simulink model "Model_silnika2"  (R2018a)
settings: Solver=ode45  StartTime=0.0  StopTime=600  FixedStep=1  MaxStep=0.004  RelTol=1e-8  EnableMultiTasking=on
values from neighbouring files (symbols this model uses):
  G = 4.2    [net_opuznienie_30.mat]    (also in parametrySilnika.m)
  J = 1    [net_opuznienie_30.mat]    (also in parametrySilnika.m)
  Lt = 46    [net_opuznienie_30.mat]    (also in parametrySilnika.m)
  Lw = 125    [net_opuznienie_30.mat]    (also in parametrySilnika.m)
  Rt = 5    [net_opuznienie_30.mat]    (also in parametrySilnika.m)
undefined symbols (not defined in the file or in its folder): sigbuilder_block
libraries: neural x22, simulink x2
(part 2 of 3)

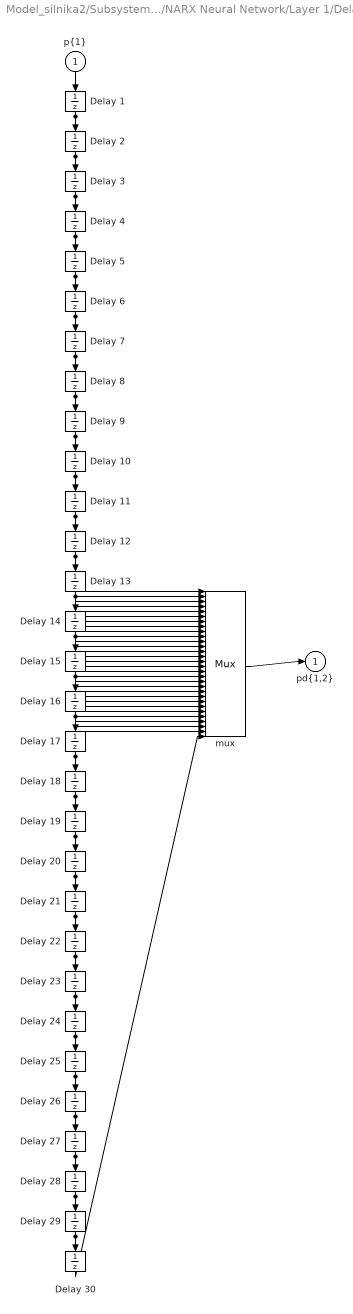
== system Model_silnika2/Subsystem/NARX Neural Network/Layer 1/Delays 2 ==
  "p{1}" : Inport  PortDimensions=3  SampleTime=0.1
      mask Display: e = 0.06;c1 = [120 230 180]/255;c2 = ([120 230 180]+0)/(256+128);c3 = ([120 230 180]+128)/(256+128);patch([0 1 1 0],[0 0 1 1],c1);patch([0 1 1 1-e 1-e 0+e],[0 0 1 1-e 0+e 0+e],c2);patch([0 0 1 1-e 0+e 0+e],[0 1 1 1-e 1-e 0+e],c3);plot([0 1 1 0 0],[0 0 1 1 0]);
  Delay 1 : UnitDelay  InitialCondition=pi_input_2_delayed_1  SampleTime=0.1
      mask Display: e = 0.06;c1 = [120 150 230]/255;c2 = ([120 150 230]+0)/383;c3 = ([120 150 230]+128)/383;patch([0 1 1 0],[0 0 1 1],c1);patch([0 1 1 1-e 1-e 0+e],[0 0 1 1-e 0+e 0+e],c2);patch([0 0 1 1-e 0+e 0+e],[0 1 1 1-e 1-e 0+e],c3);plot([0 1 1 0 0],[0 0 1 1 0]);disp('D')
  Delay 10 : UnitDelay  InitialCondition=pi_input_2_delayed_10  SampleTime=0.1
      mask Display: e = 0.06;c1 = [120 150 230]/255;c2 = ([120 150 230]+0)/383;c3 = ([120 150 230]+128)/383;patch([0 1 1 0],[0 0 1 1],c1);patch([0 1 1 1-e 1-e 0+e],[0 0 1 1-e 0+e 0+e],c2);patch([0 0 1 1-e 0+e 0+e],[0 1 1 1-e 1-e 0+e],c3);plot([0 1 1 0 0],[0 0 1 1 0]);disp('D')
  Delay 11 : UnitDelay  InitialCondition=pi_input_2_delayed_11  SampleTime=0.1
      mask Display: e = 0.06;c1 = [120 150 230]/255;c2 = ([120 150 230]+0)/383;c3 = ([120 150 230]+128)/383;patch([0 1 1 0],[0 0 1 1],c1);patch([0 1 1 1-e 1-e 0+e],[0 0 1 1-e 0+e 0+e],c2);patch([0 0 1 1-e 0+e 0+e],[0 1 1 1-e 1-e 0+e],c3);plot([0 1 1 0 0],[0 0 1 1 0]);disp('D')
  Delay 12 : UnitDelay  InitialCondition=pi_input_2_delayed_12  SampleTime=0.1
      mask Display: e = 0.06;c1 = [120 150 230]/255;c2 = ([120 150 230]+0)/383;c3 = ([120 150 230]+128)/383;patch([0 1 1 0],[0 0 1 1],c1);patch([0 1 1 1-e 1-e 0+e],[0 0 1 1-e 0+e 0+e],c2);patch([0 0 1 1-e 0+e 0+e],[0 1 1 1-e 1-e 0+e],c3);plot([0 1 1 0 0],[0 0 1 1 0]);disp('D')
  Delay 13 : UnitDelay  InitialCondition=pi_input_2_delayed_13  SampleTime=0.1
      mask Display: e = 0.06;c1 = [120 150 230]/255;c2 = ([120 150 230]+0)/383;c3 = ([120 150 230]+128)/383;patch([0 1 1 0],[0 0 1 1],c1);patch([0 1 1 1-e 1-e 0+e],[0 0 1 1-e 0+e 0+e],c2);patch([0 0 1 1-e 0+e 0+e],[0 1 1 1-e 1-e 0+e],c3);plot([0 1 1 0 0],[0 0 1 1 0]);disp('D')
  Delay 14 : UnitDelay  InitialCondition=pi_input_2_delayed_14  SampleTime=0.1
      mask Display: e = 0.06;c1 = [120 150 230]/255;c2 = ([120 150 230]+0)/383;c3 = ([120 150 230]+128)/383;patch([0 1 1 0],[0 0 1 1],c1);patch([0 1 1 1-e 1-e 0+e],[0 0 1 1-e 0+e 0+e],c2);patch([0 0 1 1-e 0+e 0+e],[0 1 1 1-e 1-e 0+e],c3);plot([0 1 1 0 0],[0 0 1 1 0]);disp('D')
  Delay 15 : UnitDelay  InitialCondition=pi_input_2_delayed_15  SampleTime=0.1
      mask Display: e = 0.06;c1 = [120 150 230]/255;c2 = ([120 150 230]+0)/383;c3 = ([120 150 230]+128)/383;patch([0 1 1 0],[0 0 1 1],c1);patch([0 1 1 1-e 1-e 0+e],[0 0 1 1-e 0+e 0+e],c2);patch([0 0 1 1-e 0+e 0+e],[0 1 1 1-e 1-e 0+e],c3);plot([0 1 1 0 0],[0 0 1 1 0]);disp('D')
  Delay 16 : UnitDelay  InitialCondition=pi_input_2_delayed_16  SampleTime=0.1
      mask Display: e = 0.06;c1 = [120 150 230]/255;c2 = ([120 150 230]+0)/383;c3 = ([120 150 230]+128)/383;patch([0 1 1 0],[0 0 1 1],c1);patch([0 1 1 1-e 1-e 0+e],[0 0 1 1-e 0+e 0+e],c2);patch([0 0 1 1-e 0+e 0+e],[0 1 1 1-e 1-e 0+e],c3);plot([0 1 1 0 0],[0 0 1 1 0]);disp('D')
  Delay 17 : UnitDelay  InitialCondition=pi_input_2_delayed_17  SampleTime=0.1
      mask Display: e = 0.06;c1 = [120 150 230]/255;c2 = ([120 150 230]+0)/383;c3 = ([120 150 230]+128)/383;patch([0 1 1 0],[0 0 1 1],c1);patch([0 1 1 1-e 1-e 0+e],[0 0 1 1-e 0+e 0+e],c2);patch([0 0 1 1-e 0+e 0+e],[0 1 1 1-e 1-e 0+e],c3);plot([0 1 1 0 0],[0 0 1 1 0]);disp('D')
  Delay 18 : UnitDelay  InitialCondition=pi_input_2_delayed_18  SampleTime=0.1
      mask Display: e = 0.06;c1 = [120 150 230]/255;c2 = ([120 150 230]+0)/383;c3 = ([120 150 230]+128)/383;patch([0 1 1 0],[0 0 1 1],c1);patch([0 1 1 1-e 1-e 0+e],[0 0 1 1-e 0+e 0+e],c2);patch([0 0 1 1-e 0+e 0+e],[0 1 1 1-e 1-e 0+e],c3);plot([0 1 1 0 0],[0 0 1 1 0]);disp('D')
  Delay 19 : UnitDelay  InitialCondition=pi_input_2_delayed_19  SampleTime=0.1
      mask Display: e = 0.06;c1 = [120 150 230]/255;c2 = ([120 150 230]+0)/383;c3 = ([120 150 230]+128)/383;patch([0 1 1 0],[0 0 1 1],c1);patch([0 1 1 1-e 1-e 0+e],[0 0 1 1-e 0+e 0+e],c2);patch([0 0 1 1-e 0+e 0+e],[0 1 1 1-e 1-e 0+e],c3);plot([0 1 1 0 0],[0 0 1 1 0]);disp('D')
  Delay 2 : UnitDelay  InitialCondition=pi_input_2_delayed_2  SampleTime=0.1
      mask Display: e = 0.06;c1 = [120 150 230]/255;c2 = ([120 150 230]+0)/383;c3 = ([120 150 230]+128)/383;patch([0 1 1 0],[0 0 1 1],c1);patch([0 1 1 1-e 1-e 0+e],[0 0 1 1-e 0+e 0+e],c2);patch([0 0 1 1-e 0+e 0+e],[0 1 1 1-e 1-e 0+e],c3);plot([0 1 1 0 0],[0 0 1 1 0]);disp('D')
  Delay 20 : UnitDelay  InitialCondition=pi_input_2_delayed_20  SampleTime=0.1
      mask Display: e = 0.06;c1 = [120 150 230]/255;c2 = ([120 150 230]+0)/383;c3 = ([120 150 230]+128)/383;patch([0 1 1 0],[0 0 1 1],c1);patch([0 1 1 1-e 1-e 0+e],[0 0 1 1-e 0+e 0+e],c2);patch([0 0 1 1-e 0+e 0+e],[0 1 1 1-e 1-e 0+e],c3);plot([0 1 1 0 0],[0 0 1 1 0]);disp('D')
  Delay 21 : UnitDelay  InitialCondition=pi_input_2_delayed_21  SampleTime=0.1
      mask Display: e = 0.06;c1 = [120 150 230]/255;c2 = ([120 150 230]+0)/383;c3 = ([120 150 230]+128)/383;patch([0 1 1 0],[0 0 1 1],c1);patch([0 1 1 1-e 1-e 0+e],[0 0 1 1-e 0+e 0+e],c2);patch([0 0 1 1-e 0+e 0+e],[0 1 1 1-e 1-e 0+e],c3);plot([0 1 1 0 0],[0 0 1 1 0]);disp('D')
  Delay 22 : UnitDelay  InitialCondition=pi_input_2_delayed_22  SampleTime=0.1
      mask Display: e = 0.06;c1 = [120 150 230]/255;c2 = ([120 150 230]+0)/383;c3 = ([120 150 230]+128)/383;patch([0 1 1 0],[0 0 1 1],c1);patch([0 1 1 1-e 1-e 0+e],[0 0 1 1-e 0+e 0+e],c2);patch([0 0 1 1-e 0+e 0+e],[0 1 1 1-e 1-e 0+e],c3);plot([0 1 1 0 0],[0 0 1 1 0]);disp('D')
  Delay 23 : UnitDelay  InitialCondition=pi_input_2_delayed_23  SampleTime=0.1
      mask Display: e = 0.06;c1 = [120 150 230]/255;c2 = ([120 150 230]+0)/383;c3 = ([120 150 230]+128)/383;patch([0 1 1 0],[0 0 1 1],c1);patch([0 1 1 1-e 1-e 0+e],[0 0 1 1-e 0+e 0+e],c2);patch([0 0 1 1-e 0+e 0+e],[0 1 1 1-e 1-e 0+e],c3);plot([0 1 1 0 0],[0 0 1 1 0]);disp('D')
  Delay 24 : UnitDelay  InitialCondition=pi_input_2_delayed_24  SampleTime=0.1
      mask Display: e = 0.06;c1 = [120 150 230]/255;c2 = ([120 150 230]+0)/383;c3 = ([120 150 230]+128)/383;patch([0 1 1 0],[0 0 1 1],c1);patch([0 1 1 1-e 1-e 0+e],[0 0 1 1-e 0+e 0+e],c2);patch([0 0 1 1-e 0+e 0+e],[0 1 1 1-e 1-e 0+e],c3);plot([0 1 1 0 0],[0 0 1 1 0]);disp('D')
  Delay 25 : UnitDelay  InitialCondition=pi_input_2_delayed_25  SampleTime=0.1
      mask Display: e = 0.06;c1 = [120 150 230]/255;c2 = ([120 150 230]+0)/383;c3 = ([120 150 230]+128)/383;patch([0 1 1 0],[0 0 1 1],c1);patch([0 1 1 1-e 1-e 0+e],[0 0 1 1-e 0+e 0+e],c2);patch([0 0 1 1-e 0+e 0+e],[0 1 1 1-e 1-e 0+e],c3);plot([0 1 1 0 0],[0 0 1 1 0]);disp('D')
  Delay 26 : UnitDelay  InitialCondition=pi_input_2_delayed_26  SampleTime=0.1
      mask Display: e = 0.06;c1 = [120 150 230]/255;c2 = ([120 150 230]+0)/383;c3 = ([120 150 230]+128)/383;patch([0 1 1 0],[0 0 1 1],c1);patch([0 1 1 1-e 1-e 0+e],[0 0 1 1-e 0+e 0+e],c2);patch([0 0 1 1-e 0+e 0+e],[0 1 1 1-e 1-e 0+e],c3);plot([0 1 1 0 0],[0 0 1 1 0]);disp('D')
  Delay 27 : UnitDelay  InitialCondition=pi_input_2_delayed_27  SampleTime=0.1
      mask Display: e = 0.06;c1 = [120 150 230]/255;c2 = ([120 150 230]+0)/383;c3 = ([120 150 230]+128)/383;patch([0 1 1 0],[0 0 1 1],c1);patch([0 1 1 1-e 1-e 0+e],[0 0 1 1-e 0+e 0+e],c2);patch([0 0 1 1-e 0+e 0+e],[0 1 1 1-e 1-e 0+e],c3);plot([0 1 1 0 0],[0 0 1 1 0]);disp('D')
  Delay 28 : UnitDelay  InitialCondition=pi_input_2_delayed_28  SampleTime=0.1
      mask Display: e = 0.06;c1 = [120 150 230]/255;c2 = ([120 150 230]+0)/383;c3 = ([120 150 230]+128)/383;patch([0 1 1 0],[0 0 1 1],c1);patch([0 1 1 1-e 1-e 0+e],[0 0 1 1-e 0+e 0+e],c2);patch([0 0 1 1-e 0+e 0+e],[0 1 1 1-e 1-e 0+e],c3);plot([0 1 1 0 0],[0 0 1 1 0]);disp('D')
  Delay 29 : UnitDelay  InitialCondition=pi_input_2_delayed_29  SampleTime=0.1
      mask Display: e = 0.06;c1 = [120 150 230]/255;c2 = ([120 150 230]+0)/383;c3 = ([120 150 230]+128)/383;patch([0 1 1 0],[0 0 1 1],c1);patch([0 1 1 1-e 1-e 0+e],[0 0 1 1-e 0+e 0+e],c2);patch([0 0 1 1-e 0+e 0+e],[0 1 1 1-e 1-e 0+e],c3);plot([0 1 1 0 0],[0 0 1 1 0]);disp('D')
  Delay 3 : UnitDelay  InitialCondition=pi_input_2_delayed_3  SampleTime=0.1
      mask Display: e = 0.06;c1 = [120 150 230]/255;c2 = ([120 150 230]+0)/383;c3 = ([120 150 230]+128)/383;patch([0 1 1 0],[0 0 1 1],c1);patch([0 1 1 1-e 1-e 0+e],[0 0 1 1-e 0+e 0+e],c2);patch([0 0 1 1-e 0+e 0+e],[0 1 1 1-e 1-e 0+e],c3);plot([0 1 1 0 0],[0 0 1 1 0]);disp('D')
  Delay 30 : UnitDelay  InitialCondition=pi_input_2_delayed_30  SampleTime=0.1
      mask Display: e = 0.06;c1 = [120 150 230]/255;c2 = ([120 150 230]+0)/383;c3 = ([120 150 230]+128)/383;patch([0 1 1 0],[0 0 1 1],c1);patch([0 1 1 1-e 1-e 0+e],[0 0 1 1-e 0+e 0+e],c2);patch([0 0 1 1-e 0+e 0+e],[0 1 1 1-e 1-e 0+e],c3);plot([0 1 1 0 0],[0 0 1 1 0]);disp('D')
  Delay 4 : UnitDelay  InitialCondition=pi_input_2_delayed_4  SampleTime=0.1
      mask Display: e = 0.06;c1 = [120 150 230]/255;c2 = ([120 150 230]+0)/383;c3 = ([120 150 230]+128)/383;patch([0 1 1 0],[0 0 1 1],c1);patch([0 1 1 1-e 1-e 0+e],[0 0 1 1-e 0+e 0+e],c2);patch([0 0 1 1-e 0+e 0+e],[0 1 1 1-e 1-e 0+e],c3);plot([0 1 1 0 0],[0 0 1 1 0]);disp('D')
  Delay 5 : UnitDelay  InitialCondition=pi_input_2_delayed_5  SampleTime=0.1
      mask Display: e = 0.06;c1 = [120 150 230]/255;c2 = ([120 150 230]+0)/383;c3 = ([120 150 230]+128)/383;patch([0 1 1 0],[0 0 1 1],c1);patch([0 1 1 1-e 1-e 0+e],[0 0 1 1-e 0+e 0+e],c2);patch([0 0 1 1-e 0+e 0+e],[0 1 1 1-e 1-e 0+e],c3);plot([0 1 1 0 0],[0 0 1 1 0]);disp('D')
  Delay 6 : UnitDelay  InitialCondition=pi_input_2_delayed_6  SampleTime=0.1
      mask Display: e = 0.06;c1 = [120 150 230]/255;c2 = ([120 150 230]+0)/383;c3 = ([120 150 230]+128)/383;patch([0 1 1 0],[0 0 1 1],c1);patch([0 1 1 1-e 1-e 0+e],[0 0 1 1-e 0+e 0+e],c2);patch([0 0 1 1-e 0+e 0+e],[0 1 1 1-e 1-e 0+e],c3);plot([0 1 1 0 0],[0 0 1 1 0]);disp('D')
  Delay 7 : UnitDelay  InitialCondition=pi_input_2_delayed_7  SampleTime=0.1
      mask Display: e = 0.06;c1 = [120 150 230]/255;c2 = ([120 150 230]+0)/383;c3 = ([120 150 230]+128)/383;patch([0 1 1 0],[0 0 1 1],c1);patch([0 1 1 1-e 1-e 0+e],[0 0 1 1-e 0+e 0+e],c2);patch([0 0 1 1-e 0+e 0+e],[0 1 1 1-e 1-e 0+e],c3);plot([0 1 1 0 0],[0 0 1 1 0]);disp('D')
  Delay 8 : UnitDelay  InitialCondition=pi_input_2_delayed_8  SampleTime=0.1
      mask Display: e = 0.06;c1 = [120 150 230]/255;c2 = ([120 150 230]+0)/383;c3 = ([120 150 230]+128)/383;patch([0 1 1 0],[0 0 1 1],c1);patch([0 1 1 1-e 1-e 0+e],[0 0 1 1-e 0+e 0+e],c2);patch([0 0 1 1-e 0+e 0+e],[0 1 1 1-e 1-e 0+e],c3);plot([0 1 1 0 0],[0 0 1 1 0]);disp('D')
  Delay 9 : UnitDelay  InitialCondition=pi_input_2_delayed_9  SampleTime=0.1
      mask Display: e = 0.06;c1 = [120 150 230]/255;c2 = ([120 150 230]+0)/383;c3 = ([120 150 230]+128)/383;patch([0 1 1 0],[0 0 1 1],c1);patch([0 1 1 1-e 1-e 0+e],[0 0 1 1-e 0+e 0+e],c2);patch([0 0 1 1-e 0+e 0+e],[0 1 1 1-e 1-e 0+e],c3);plot([0 1 1 0 0],[0 0 1 1 0]);disp('D')
  mux : Mux  Inputs=30
      mask Display: e = 0.06;c1 = [120 150 230]/255;c2 = ([120 150 230]+0)/383;c3 = ([120 150 230]+128)/383;patch([0 1 1 0],[0 0 1 1],c1);patch([0 1 1 1-e 1-e 0+e],[0 0 1 1-e 0+e 0+e],c2);patch([0 0 1 1-e 0+e 0+e],[0 1 1 1-e 1-e 0+e],c3);plot([0 1 1 0 0],[0 0 1 1 0]);disp('Mux')
  "pd{1,2}" : Outport
      mask Display: e = 0.06;c1 = [120 230 180]/255;c2 = ([120 230 180]+0)/(256+128);c3 = ([120 230 180]+128)/(256+128);patch([0 1 1 0],[0 0 1 1],c1);patch([0 1 1 1-e 1-e 0+e],[0 0 1 1-e 0+e 0+e],c2);patch([0 0 1 1-e 0+e 0+e],[0 1 1 1-e 1-e 0+e],c3);plot([0 1 1 0 0],[0 0 1 1 0]);
  wires:
  "p{1}"/1 -> Delay 1/1
  Delay 1/1 -> Delay 2/1, mux/1
  Delay 2/1 -> Delay 3/1, mux/2
  Delay 3/1 -> Delay 4/1, mux/3
  Delay 4/1 -> Delay 5/1, mux/4
  Delay 5/1 -> Delay 6/1, mux/5
  Delay 6/1 -> Delay 7/1, mux/6
  Delay 7/1 -> Delay 8/1, mux/7
  Delay 8/1 -> Delay 9/1, mux/8
  Delay 9/1 -> Delay 10/1, mux/9
  Delay 10/1 -> Delay 11/1, mux/10
  Delay 11/1 -> Delay 12/1, mux/11
  Delay 12/1 -> Delay 13/1, mux/12
  Delay 13/1 -> Delay 14/1, mux/13
  Delay 14/1 -> Delay 15/1, mux/14
  Delay 15/1 -> Delay 16/1, mux/15
  Delay 16/1 -> Delay 17/1, mux/16
  Delay 17/1 -> Delay 18/1, mux/17
  Delay 18/1 -> Delay 19/1, mux/18
  Delay 19/1 -> Delay 20/1, mux/19
  Delay 20/1 -> Delay 21/1, mux/20
  Delay 21/1 -> Delay 22/1, mux/21
  Delay 22/1 -> Delay 23/1, mux/22
  Delay 23/1 -> Delay 24/1, mux/23
  Delay 24/1 -> Delay 25/1, mux/24
  Delay 25/1 -> Delay 26/1, mux/25
  Delay 26/1 -> Delay 27/1, mux/26
  Delay 27/1 -> Delay 28/1, mux/27
  Delay 28/1 -> Delay 29/1, mux/28
  Delay 29/1 -> Delay 30/1, mux/29
  Delay 30/1 -> mux/30
  mux/1 -> "pd{1,2}"/1

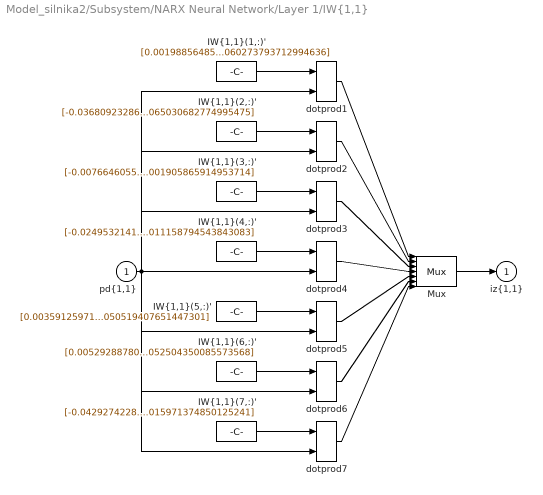
== system Model_silnika2/Subsystem/NARX Neural Network/Layer 1/IW{1,1} ==
  "pd{1,1}" : Inport  PortDimensions=93  SampleTime=0.1
      mask Display: e = 0.06;c1 = [120 230 180]/255;c2 = ([120 230 180]+0)/(256+128);c3 = ([120 230 180]+128)/(256+128);patch([0 1 1 0],[0 0 1 1],c1);patch([0 1 1 1-e 1-e 0+e],[0 0 1 1-e 0+e 0+e],c2);patch([0 0 1 1-e 0+e 0+e],[0 1 1 1-e 1-e 0+e],c3);plot([0 1 1 0 0],[0 0 1 1 0]);
  "IW{1,1}(1,:)'" : Constant  Value=[0.0019885648572870711;0.00017353216044262241;0.00020246318392944663;0.0012877889136962829;0.0041621575399698862;0.004146431914045119;0.0031122554266859951;0.0072578529035021563;0.007221608539589231;0.0052886978249656455;0.0096265541469795594;0.0096097866153640188;0.0037072305592038514;0.010159213000665725;0.010153021947951481;0.0020284555667614071;0.0094199191911381822;0.0094369659993983907;0.0022816816539381404;0.0071232650382990906;0.0071537518067209304;0.0016626187475556919;0.0047518269829249444;0.0047531056147696706;0.0020121305033980598;0.0025672373543122948;0.002577118947758473;0.0034272863518573196;0.00016888799192580465;0.00018905384494078149;0.0037618836764962589;-0.0018604907625631168;-0.0018757218477068655;0.0067485305203867987;-0.0033535570623899873;-0.0033435156926478133;0.0064292299509081932;-0.0049475392854431534;-0.0049515590045061068;0.0091330520987752805;-0.0058607117799318615;-0.0058645572190691719;0.0097185636515801262;-0.0063177974309289201;-0.0062841625672411484;0.011049853079969906;-0.0066066019753691129;-0.00660886754201713;0.011639652187494744;-0.0058638683193952866;-0.0058674765812183555;0.012277307839238506;-0.0062434092143199308;-0.006223173999384257;0.012184300722183823;-0.0049910581364777896;-0.0049602741139057847;0.012369523833305114;-0.0040177057475507556;-0.0040258670882894884;0.012707114686688135;-0.0031374496005083527;-0.0031135632071982462;0.01199815190430247;-0.0014803465930950306;-0.0014817157917846025;0.011745661192756328;-0.00013594683155318063;-0.00012740864850212361;0.012929416864156986;0.00094004208381961172;0.00096521495097527221;0.012502965348679465;0.0023279754869333273;0.0023414545896575357;0.012482435998225856;0.0035419671709262944;0.0035762178877970798;0.011934548300930431;0.0053325738868501282;0.0053320827850480155;0.013046636614108929;0.0062096453902115182;0.0062246560250742529;0.011663539355452375;0.0064304649638875439;0.0064084155992088186;0.010450554421592198;0.0061677203783633708;0.0061797856121988005;0.011067516086346763;0.0060248674964442734;0.0060273793712994636]
      mask Display: e = 0.06;c1 = [120 150 230]/255;c2 = ([120 150 230]+0)/383;c3 = ([120 150 230]+128)/383;patch([0 1 1 0],[0 0 1 1],c1);patch([0 1 1 1-e 1-e 0+e],[0 0 1 1-e 0+e 0+e],c2);patch([0 0 1 1-e 0+e 0+e],[0 1 1 1-e 1-e 0+e],c3);plot([0 1 1 0 0],[0 0 1 1 0]);disp('Weights');
  "IW{1,1}(2,:)'" : Constant  Value=[-0.03680923286623293;0.025215958210341321;0.025191876987067676;-0.034153384448485612;0.024063629556723632;0.02404265159227895;-0.030487212660508366;0.022144925280749239;0.022106187781516771;-0.026859037089298522;0.019689245268806482;0.019715780530329522;-0.02468526855312566;0.016516588171180301;0.016524213109626922;-0.022695789377278296;0.012715426366594689;0.012752544524029415;-0.020156834591642563;0.0083737663442279859;0.008377356952699113;-0.01792882104581392;0.003963595507632851;0.0039637470964308946;-0.01498767046199004;-4.9456871022110553e-05;-7.9445729385161992e-05;-0.011372105946886809;-0.0035765479627977502;-0.0035923381340926702;-0.0079894622040690734;-0.0066533549247146948;-0.0066203605988653397;-0.004043202763429384;-0.0089192912789356742;-0.0088909998267149709;-0.001375045309514116;-0.011229821222691011;-0.011233430056455107;0.0020227825901768999;-0.012859892709453988;-0.012861008152047815;0.0048546825941336831;-0.01383926836744738;-0.013829553396572589;0.0072545813229751262;-0.014533696655662112;-0.014547831275745167;0.0089438640831206399;-0.01445291075726691;-0.014456316411346329;0.010370767359619755;-0.014669870337057684;-0.014666959249565592;0.011051647416366481;-0.013851038859060147;-0.013854928157819064;0.011414804606182162;-0.013440498542700576;-0.013437280320999244;0.011817958426225416;-0.013077862131358578;-0.013085944535545744;0.011889264426307739;-0.012151921817595127;-0.012152494578213956;0.011803270873627833;-0.011293556937451647;-0.011270072938144112;0.011858328407325773;-0.010430807682652582;-0.010431336347693823;0.011339670981287958;-0.0094576249475570254;-0.0094426100981729894;0.011057000374518903;-0.0086155962492994662;-0.0086540404890446624;0.0099484260683701687;-0.0076154062550492672;-0.007594172765159223;0.009014773366731399;-0.0069859248919153065;-0.0069986384129998701;0.0066053208315398244;-0.0067985909291236029;-0.0067978012725416559;0.0044751367755976202;-0.0067350110232024911;-0.0067473465466301886;0.0041511708943185247;-0.006514042265822589;-0.0065030682774995475]
      mask Display: e = 0.06;c1 = [120 150 230]/255;c2 = ([120 150 230]+0)/383;c3 = ([120 150 230]+128)/383;patch([0 1 1 0],[0 0 1 1],c1);patch([0 1 1 1-e 1-e 0+e],[0 0 1 1-e 0+e 0+e],c2);patch([0 0 1 1-e 0+e 0+e],[0 1 1 1-e 1-e 0+e],c3);plot([0 1 1 0 0],[0 0 1 1 0]);disp('Weights');
  "IW{1,1}(3,:)'" : Constant  Value=[-0.0076646055777691447;0.0070763234502732838;0.0070842203536176764;-0.004594913111176613;0.00038964116521432435;0.00041137158750551158;-0.0055103091263933625;-0.0049698101367087431;-0.0049412877899630211;-0.0075325442099127291;-0.0095426577629565013;-0.0095450227927753265;-0.0060297870176984304;-0.01209467695642937;-0.012105590036045317;-0.0044564633847823439;-0.012815090396055499;-0.012833693489322106;-0.0050632626749825185;-0.011506247072813098;-0.011504150966507259;-0.0041971286806833982;-0.0099695988637943291;-0.0099425354167575215;-0.0047297180263328863;-0.0082225182406181346;-0.0082109420612531767;-0.0067358883907070741;-0.0059865998064806223;-0.0059684859614520733;-0.0074868297025780604;-0.0040227287991187544;-0.0040515110992039843;-0.011732321752348762;-0.002409628897517291;-0.0024049134196149312;-0.012627903895818169;-0.00053672640906698055;-0.0005716310236179667;-0.016835849365649313;0.00086902971839981815;0.00087478298754549986;-0.018940044323451959;0.0017801611802645415;0.0018173051495409172;-0.02200354703831504;0.0025552877957088988;0.002585355729384693;-0.024609533244623949;0.0024114075415604687;0.0023826032603090465;-0.027037040480159313;0.0035213804790525938;0.0035144012931958468;-0.028721304805968094;0.0029288786376778907;0.0029422387894351893;-0.030291298317651628;0.0028880625472197555;0.0028814799615048377;-0.032013383924733345;0.00300445969541639;0.0030064049406744548;-0.031671424258573944;0.0022868466292456638;0.0023006048521897796;-0.031286120167063426;0.0017743262488769227;0.001774390100282909;-0.031572071293566019;0.0013442866037685151;0.0013360455361241812;-0.030039011394857935;0.00067713247476120387;0.0006818199996063125;-0.02884953861886283;0.00018619370936413836;0.00018991909697096154;-0.026606256381875752;-0.00086325294604902277;-0.00083595550254723428;-0.026549482570305025;-0.0010631146031886639;-0.0010670006856293985;-0.024506533022186059;-0.00043396403427776043;-0.00043993942798726393;-0.023857218832608072;0.00077160857113643981;0.00076178553565276071;-0.027315974330495405;0.0019114969343765071;0.001905865914953714]
      mask Display: e = 0.06;c1 = [120 150 230]/255;c2 = ([120 150 230]+0)/383;c3 = ([120 150 230]+128)/383;patch([0 1 1 0],[0 0 1 1],c1);patch([0 1 1 1-e 1-e 0+e],[0 0 1 1-e 0+e 0+e],c2);patch([0 0 1 1-e 0+e 0+e],[0 1 1 1-e 1-e 0+e],c3);plot([0 1 1 0 0],[0 0 1 1 0]);disp('Weights');
  "IW{1,1}(4,:)'" : Constant  Value=[-0.024953214152112446;0.017578647700541843;0.017608634271546918;-0.025588820938720846;0.014549255924575141;0.014550126941371457;-0.026417842514427088;0.01147470305506669;0.011445717308638288;-0.026961255328549059;0.0082363745066816631;0.0082013756291282516;-0.027018906125422449;0.005036783567107927;0.0050678034015124015;-0.026671111694633067;0.0022447302008953103;0.0022171969117303798;-0.026090237135677489;-0.00017533098161182927;-0.00019018529225397281;-0.025134837113502468;-0.0024871079659541965;-0.0024828696492451936;-0.023782095946141415;-0.004256367260575834;-0.0042656632777644124;-0.022130683470411014;-0.0053444351789336889;-0.005366701687299873;-0.020277090535669787;-0.0061031946592581916;-0.0060891997791776139;-0.018839830214806216;-0.006223231525543332;-0.0062156093638447672;-0.017268371700014457;-0.0062377253661623742;-0.0062643243250359642;-0.01625675960138679;-0.0057526015649238208;-0.0057310847803064627;-0.015211110193193092;-0.0049240319469992643;-0.0049306795812584748;-0.01463586456630382;-0.0039976779854303066;-0.0040410249695505595;-0.014635588838467288;-0.0028053020014475534;-0.0027980922398539877;-0.014750113931144775;-0.0015177271525010441;-0.0014799942746023087;-0.015234792103127927;-0.00010261601384378528;-8.7029409396311919e-05;-0.015998182674261625;0.0011597321065536339;0.001143829433398573;-0.016649131067453686;0.0022598269028675584;0.0022387278018720495;-0.016732540974371306;0.0033678647677113948;0.003376795470470398;-0.016903766148265997;0.0043405711349634116;0.0043066270239116595;-0.016981130992204024;0.0051828859263470788;0.0051571659249885909;-0.01664508850628334;0.0060185665848738685;0.0060070480999806523;-0.016048505280874117;0.0067545034454371908;0.0067220477720790414;-0.015167167099549997;0.0075096471932779687;0.0074816815870082489;-0.01427165616158326;0.008121188999079855;0.0081210376691659963;-0.01301693526491484;0.0088954088064422867;0.008884273434918705;-0.011429650812850183;0.0098725597150395843;0.0098790844536994563;-0.0099670414762932959;0.011129666809469901;0.011158794543843083]
      mask Display: e = 0.06;c1 = [120 150 230]/255;c2 = ([120 150 230]+0)/383;c3 = ([120 150 230]+128)/383;patch([0 1 1 0],[0 0 1 1],c1);patch([0 1 1 1-e 1-e 0+e],[0 0 1 1-e 0+e 0+e],c2);patch([0 0 1 1-e 0+e 0+e],[0 1 1 1-e 1-e 0+e],c3);plot([0 1 1 0 0],[0 0 1 1 0]);disp('Weights');
  "IW{1,1}(5,:)'" : Constant  Value=[0.0035912597198759478;0.0022194699294250204;0.0022070743640280372;0.00077847037868036687;0.0050083939769279264;0.0050228843958537196;-0.00025144755070802613;0.0071198457217213169;0.0071415387697813327;-0.00086180715771119287;0.0087201391749727984;0.0087414817602086588;-0.0031340365905234624;0.0092886883037458876;0.0092873220168890082;-0.0052954704366534296;0.0088471957109749807;0.0088259433338954574;-0.0065829532588685333;0.0072713864638687276;0.0072987417680781368;-0.0083163026255622594;0.0055368028928486843;0.0055199532455692518;-0.0097112289078713759;0.0035529734453227432;0.0035518652840302524;-0.010591020446259088;0.0013446741432513892;0.0013416992132362008;-0.011913605031789351;-0.0007186430117100544;-0.00071908121405710667;-0.011919892468382548;-0.0025882079972884874;-0.0025620137884845794;-0.013590094113028929;-0.0045526144512863503;-0.0045560491431301522;-0.013689563681360661;-0.0061740946442150283;-0.0061594999080722447;-0.014656779881288169;-0.0073538128567747956;-0.0073736306015660513;-0.015263638500944492;-0.0083611992289845533;-0.0083598034601088615;-0.015908944896438883;-0.0086414553497181565;-0.0086474989103364642;-0.016518718019227187;-0.0093603927472191498;-0.0093492063584030456;-0.017515304931307096;-0.0089816009426515013;-0.0089807669944180959;-0.018270911741919794;-0.0087790443042900703;-0.0087976678334840894;-0.01906235024901845;-0.008437788654195073;-0.0084384877720136888;-0.020472522250278725;-0.0074866456040048792;-0.0074933545891612847;-0.021479409476140545;-0.0064436338273677089;-0.0064192896558623843;-0.021732519527068981;-0.0051706023148107875;-0.0051875565808949852;-0.02259147221813064;-0.0037285928810473321;-0.0037182858034055443;-0.022650667293692871;-0.002192345434636608;-0.0022154630191904448;-0.023094601281733965;-0.00030963508331347282;-0.00028814305386080816;-0.021641636092181626;0.0013783285511740138;0.0014080306509820042;-0.020295486602463327;0.0027711832781927449;0.0027738717342319585;-0.016661812474125567;0.0038592662976353266;0.0038360091476565554;-0.0094662188722694392;0.0050267142573103335;0.0050519407651447301]
      mask Display: e = 0.06;c1 = [120 150 230]/255;c2 = ([120 150 230]+0)/383;c3 = ([120 150 230]+128)/383;patch([0 1 1 0],[0 0 1 1],c1);patch([0 1 1 1-e 1-e 0+e],[0 0 1 1-e 0+e 0+e],c2);patch([0 0 1 1-e 0+e 0+e],[0 1 1 1-e 1-e 0+e],c3);plot([0 1 1 0 0],[0 0 1 1 0]);disp('Weights');
  "IW{1,1}(6,:)'" : Constant  Value=[0.0052928878042780179;-0.0025753065097767853;-0.0025758051208712982;0.0068216665336466335;-0.0079511153434142293;-0.0079433138774494243;0.0057078495493609101;-0.012378658652655227;-0.012380743639209468;0.0046156340450630457;-0.016201851560737147;-0.01618743605339705;0.0078831837590174064;-0.018081756866652567;-0.01809827946408011;0.01159934545123035;-0.01847763344280005;-0.018473405265828382;0.013252498379862403;-0.017023380212477499;-0.017009733701925836;0.015914720827213152;-0.015412720805715483;-0.01543395358124736;0.017600574172222341;-0.013764240450822685;-0.013745752509640127;0.018193904364199202;-0.011563353566653084;-0.011538393863117875;0.019820170980550941;-0.0095168443909042361;-0.0095238984037360214;0.018449227249202713;-0.0077115338489178609;-0.0076874922431354586;0.020459729419441457;-0.005676412874902205;-0.0056893160741749559;0.018826627784329506;-0.0040012520828199517;-0.0040162515145911893;0.019173271711041266;-0.0026821762790689061;-0.0027130496675827902;0.018409513789265135;-0.0014402794204748438;-0.0014413806330315978;0.018026663205297513;-0.0010501623963622758;-0.0010642586981462509;0.017381241488237463;0.00051335734373339839;0.00049741751912504254;0.01722967511983332;0.00035612025725399797;0.0003445260562279895;0.016476028699224286;0.00041080424005937919;0.0004020243678237399;0.015638269128118915;0.00046075719132243105;0.00043642314891721446;0.015973155450651515;-0.00032714279874286589;-0.00034764242028909959;0.015938689727687246;-0.00095072193279640324;-0.00096108340426916128;0.014315588016341047;-0.0012697049874928199;-0.0012809286605176991;0.014720976238950722;-0.0020102789833599892;-0.001982480078496409;0.014857096641850087;-0.0025628854448713754;-0.0025963369184599417;0.015665535560852012;-0.0036848512742078589;-0.0036754759775431967;0.015091019415137085;-0.0039684954190162278;-0.0039546061928182191;0.018071039173645484;-0.0033411012621423898;-0.0033322754867473776;0.021950920824934987;-0.0020248203259637327;-0.0020060049126480947;0.024436945933773678;-0.00054154117804572951;-0.00052504350085573568]
      mask Display: e = 0.06;c1 = [120 150 230]/255;c2 = ([120 150 230]+0)/383;c3 = ([120 150 230]+128)/383;patch([0 1 1 0],[0 0 1 1],c1);patch([0 1 1 1-e 1-e 0+e],[0 0 1 1-e 0+e 0+e],c2);patch([0 0 1 1-e 0+e 0+e],[0 1 1 1-e 1-e 0+e],c3);plot([0 1 1 0 0],[0 0 1 1 0]);disp('Weights');
  "IW{1,1}(7,:)'" : Constant  Value=[-0.042927422862016056;-0.0068973966631276579;-0.0068715823115437832;-0.040104637060147365;-0.0062798856251740053;-0.0062525970079570573;-0.037424851019302229;-0.0052751803727963233;-0.0052979450752121396;-0.035021558104020654;-0.00392897485096562;-0.0039309581355113313;-0.032712646356138332;-0.002410950300443917;-0.0023958499892011388;-0.030783053644506283;-0.00077277041415505367;-0.00075227445618278213;-0.029104390966431502;0.00090516378768943468;0.00091182119868861921;-0.027594110371326624;0.0026657737066757017;0.0026662543502051794;-0.026363568704416501;0.0041958105119658364;0.0041758282611878582;-0.025627538291134188;0.0052819811516783234;0.0052873733236027207;-0.025101425026276054;0.0061808441644956979;0.0061679791545691705;-0.024575451628391101;0.0065189854029829939;0.0065156227327349912;-0.024090870940930594;0.0069066958752046275;0.0069090020461833844;-0.023513374432743744;0.006781298951322629;0.0067753807095779113;-0.022905644899780597;0.0063052760834857186;0.0062998625302003097;-0.022083597784558189;0.0056884223940976853;0.0056903073321372382;-0.0209238101860343;0.0046845450668517152;0.0046762056774133911;-0.019673453992966852;0.0036660281585210201;0.0036726915777434196;-0.017977965293646866;0.0023209219758186183;0.0023308819326905449;-0.016094170096744145;0.0011369808097285059;0.0011644704970714421;-0.014133751238946697;3.0037191845101407e-06;4.1831548592859623e-05;-0.012349091015197974;-0.0012979588981333284;-0.0012926957669873946;-0.010428506523977088;-0.0025526345086930363;-0.0025777630934945817;-0.0085438617738588293;-0.0039573061706136992;-0.0039434394200699692;-0.0068777351504184349;-0.0053511488151192846;-0.0053589909003482691;-0.0057485792812699815;-0.0067792433496771604;-0.0067677385163032316;-0.0048252463683823377;-0.0084076215650659147;-0.0083982573801398824;-0.0046856326090569476;-0.0099968979949325212;-0.0099858052512837615;-0.0055298705697105479;-0.011751416150613939;-0.011738775524895707;-0.0078475853664329298;-0.01369232921762484;-0.013702128429836946;-0.011506103022178926;-0.015948853263909893;-0.015971374850125241]
      mask Display: e = 0.06;c1 = [120 150 230]/255;c2 = ([120 150 230]+0)/383;c3 = ([120 150 230]+128)/383;patch([0 1 1 0],[0 0 1 1],c1);patch([0 1 1 1-e 1-e 0+e],[0 0 1 1-e 0+e 0+e],c2);patch([0 0 1 1-e 0+e 0+e],[0 1 1 1-e 1-e 0+e],c3);plot([0 1 1 0 0],[0 0 1 1 0]);disp('Weights');
  Mux : Mux  Inputs=7
      mask Display: e = 0.06;c1 = [120 150 230]/255;c2 = ([120 150 230]+0)/383;c3 = ([120 150 230]+128)/383;patch([0 1 1 0],[0 0 1 1],c1);patch([0 1 1 1-e 1-e 0+e],[0 0 1 1-e 0+e 0+e],c2);patch([0 0 1 1-e 0+e 0+e],[0 1 1 1-e 1-e 0+e],c3);plot([0 1 1 0 0],[0 0 1 1 0]);disp('Mux');
  dotprod{1..7} (7 alike) : neural/Weight Functions/dotprod
  "iz{1,1}" : Outport
      mask Display: e = 0.06;c1 = [120 230 180]/255;c2 = ([120 230 180]+0)/(256+128);c3 = ([120 230 180]+128)/(256+128);patch([0 1 1 0],[0 0 1 1],c1);patch([0 1 1 1-e 1-e 0+e],[0 0 1 1-e 0+e 0+e],c2);patch([0 0 1 1-e 0+e 0+e],[0 1 1 1-e 1-e 0+e],c3);plot([0 1 1 0 0],[0 0 1 1 0]);
  wires:
  "IW{1,1}(1,:)'"/1 -> dotprod1/1
  "pd{1,1}"/1 -> dotprod1/2, dotprod2/2, dotprod3/2, dotprod4/2, dotprod5/2, dotprod6/2, dotprod7/2
  dotprod1/1 -> Mux/1
  "IW{1,1}(2,:)'"/1 -> dotprod2/1
  dotprod2/1 -> Mux/2
  "IW{1,1}(3,:)'"/1 -> dotprod3/1
  dotprod3/1 -> Mux/3
  "IW{1,1}(4,:)'"/1 -> dotprod4/1
  dotprod4/1 -> Mux/4
  "IW{1,1}(5,:)'"/1 -> dotprod5/1
  dotprod5/1 -> Mux/5
  "IW{1,1}(6,:)'"/1 -> dotprod6/1
  dotprod6/1 -> Mux/6
  "IW{1,1}(7,:)'"/1 -> dotprod7/1
  dotprod7/1 -> Mux/7
  Mux/1 -> "iz{1,1}"/1

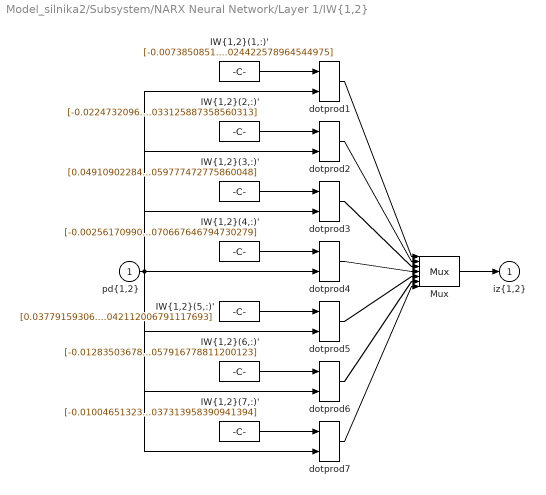
== system Model_silnika2/Subsystem/NARX Neural Network/Layer 1/IW{1,2} ==
  "pd{1,2}" : Inport  PortDimensions=90  SampleTime=0.1
      mask Display: e = 0.06;c1 = [120 230 180]/255;c2 = ([120 230 180]+0)/(256+128);c3 = ([120 230 180]+128)/(256+128);patch([0 1 1 0],[0 0 1 1],c1);patch([0 1 1 1-e 1-e 0+e],[0 0 1 1-e 0+e 0+e],c2);patch([0 0 1 1-e 0+e 0+e],[0 1 1 1-e 1-e 0+e],c3);plot([0 1 1 0 0],[0 0 1 1 0]);
  "IW{1,2}(1,:)'" : Constant  Value=[-0.0073850851884525804;-0.036481630737896023;0.059444909345194537;-0.0081166668334832822;-0.018474115313929694;0.047228591178252018;-0.0087046085461755952;-0.00548453074564576;0.036108652686082147;-0.0076653933133732323;0.0033179443692096951;0.026226601926989654;-0.0078671199084445441;0.0086582881384348279;0.017469098773388619;-0.0065550248903158068;0.011510919797171679;0.00992875545431369;-0.0057874554534784331;0.012495809393787317;0.0035549872834272416;-0.0047510827005465914;0.012055285389549057;-0.001713863297546931;-0.003038228662705571;0.010714363949111873;-0.0058693727511049754;-0.002469141570865811;0.0086157945683637445;-0.0090544809568938213;-0.0014171939878078865;0.0062295965613732808;-0.011326984166344064;-0.00049518673289645587;0.0036883924850462497;-0.01273569546603281;-0.00058430754801802034;0.001181961636954175;-0.013384860829923453;0.00060359521254734925;-0.0012039637651931714;-0.013344541419518092;0.0003422084081000178;-0.0033085373908097772;-0.012718143385728332;0.00020200654750992977;-0.0051951317122341644;-0.011550085671145217;0.00052804685584406142;-0.0067063220705424103;-0.0099625204670768606;-0.00015498119599549305;-0.007712867411429754;-0.0080056147621379772;0.00031852649912373563;-0.0084776209325578469;-0.0057842212211278877;-3.1513637335789431e-05;-0.008829010027599532;-0.0033083658454754364;-0.00039492024216146953;-0.0087041385796573362;-0.00068998928069583833;-0.0002477963117443165;-0.0082510923998185947;0.0021018542490104206;-0.0019800478104403272;-0.0073460459189140714;0.0049716642429169415;-0.0016721498614370089;-0.0058437632039834387;0.0078790067197087536;-0.0028388458835081867;-0.0035774663617792451;0.010764854904289889;-0.0054411503364246031;-0.00044380004265905917;0.013672263824571177;-0.0068124342595826236;0.0038809290987699692;0.016542286624420696;-0.010582331631717217;0.010016313490451815;0.019308850187062399;-0.013612199387408276;0.0190975288632531;0.021973076793418284;-0.018027795920275622;0.031578586495462906;0.024422578964544975]
      mask Display: e = 0.06;c1 = [120 150 230]/255;c2 = ([120 150 230]+0)/383;c3 = ([120 150 230]+128)/383;patch([0 1 1 0],[0 0 1 1],c1);patch([0 1 1 1-e 1-e 0+e],[0 0 1 1-e 0+e 0+e],c2);patch([0 0 1 1-e 0+e 0+e],[0 1 1 1-e 1-e 0+e],c3);plot([0 1 1 0 0],[0 0 1 1 0]);disp('Weights');
  "IW{1,2}(2,:)'" : Constant  Value=[-0.022473209617382587;0.062693185987088493;0.022815917477947333;-0.020340960583043959;0.055695689527969709;0.018332756937629337;-0.018124822752717252;0.04788548651351255;0.014244612758578447;-0.015331588304684299;0.03968626786574983;0.01069409689406949;-0.012921103732865674;0.031374761198548824;0.0075494939630136263;-0.0098393230495456684;0.023425286065673324;0.0049215940344426775;-0.0069929229196640198;0.016029714845060685;0.0027265306734429802;-0.0041685376397519094;0.0093958953813454062;0.00099500600154048659;-0.0012826432090384614;0.0035416967898547328;-0.00029742604007959968;0.00086487672708776347;-0.0015570777744415044;-0.0012092016945983665;0.0030548992253606566;-0.0058788262056655247;-0.0017197992264422945;0.0048688174166299806;-0.0094717105780949811;-0.001869785488887793;0.0059666582866721727;-0.012252729062714669;-0.0016997151529350323;0.0071714839648197486;-0.014347471781488073;-0.0012400185224534313;0.0076358575741393431;-0.015878066574276744;-0.00042477362785180579;0.0078977133593032996;-0.016864645130927607;0.00061296852675716185;0.0080897210246832132;-0.017297284848222638;0.0018675841555617356;0.0079237657663664904;-0.017231691434369024;0.0033743264662882424;0.0080195365322033984;-0.016706295743325248;0.0051086410319225381;0.0076657180222542472;-0.01558847641756156;0.0069865519695785734;0.0071821992211023476;-0.013883953203103929;0.00909310246677285;0.006883998067561823;-0.011634938768944903;0.011300304165160882;0.0059562915458991955;-0.0087674543404259245;0.013674524935945622;0.0055602133300582061;-0.0051594207089516141;0.016177345896681461;0.0050959854152573441;-0.00078458598612530237;0.018792064534616858;0.0040757731138599323;0.0045447473269089817;0.021530096721715377;0.0048386544542015448;0.011074624822798354;0.024364062837884417;0.0058796256454599904;0.019265216219498262;0.027231556138962255;0.0080978997107105117;0.029698961468019786;0.030169172660135576;0.01273521078642216;0.042718312855386797;0.033125887358560313]
      mask Display: e = 0.06;c1 = [120 150 230]/255;c2 = ([120 150 230]+0)/383;c3 = ([120 150 230]+128)/383;patch([0 1 1 0],[0 0 1 1],c1);patch([0 1 1 1-e 1-e 0+e],[0 0 1 1-e 0+e 0+e],c2);patch([0 0 1 1-e 0+e 0+e],[0 1 1 1-e 1-e 0+e],c3);plot([0 1 1 0 0],[0 0 1 1 0]);disp('Weights');
  "IW{1,2}(3,:)'" : Constant  Value=[0.049109022848822646;0.042692615696081217;-0.0766385526806279;0.049681101134240596;0.025197434429492727;-0.064768924200522021;0.049865350613159054;0.012331430878830001;-0.053883888958694177;0.048599959374725832;0.0032454162853449786;-0.043929490888640343;0.048390656316927162;-0.0026125408030039337;-0.034958706689799751;0.046421720015235549;-0.0063262748766389791;-0.026947441771052377;0.044885553974002124;-0.0084635964879872048;-0.019945834519150704;0.04270200389649069;-0.0093767057754024098;-0.013859576675127607;0.039884641980278773;-0.009664498837792827;-0.008679258538807107;0.037873156184991395;-0.0094208543404061332;-0.0043792178240638349;0.035443205195326698;-0.0090115714377675352;-0.00082059541918912181;0.03311271651324834;-0.0084656618005141612;0.0020277378264384246;0.031619977970696565;-0.0080195906140358292;0.0041934707425108266;0.029239964631553213;-0.007701612180952503;0.0058171170992251655;0.02803043525522898;-0.0073864984535786851;0.0069537502816319529;0.02734858878730409;-0.0070523935884071465;0.0076323036802804578;0.026231020875165777;-0.006678643077015791;0.0079057379080983304;0.02642215515924435;-0.006300369842825896;0.0078701627133142531;0.026112361572351306;-0.0055846341920407277;0.0075470323097734946;0.026303900849825958;-0.0045746539224193437;0.0069967658054776328;0.026903008889918593;-0.0032176447695864154;0.0062555461274214014;0.026552675410020338;-0.0013228626584585966;0.0053754300003269941;0.027369232790254938;0.00099630991317606983;0.0042746404073453368;0.025872187473941825;0.0035952925457740426;0.0030785066458867611;0.023616348341230678;0.0062821688829581149;0.0017328578728776514;0.021562973109748383;0.0086759759553607339;0.00030394868493266881;0.015867040155365629;0.010286570914273532;-0.0012112565266805839;0.0085879453807074738;0.010193448426597336;-0.0027706692554555902;-0.0012198291840922614;0.0068219791885781459;-0.0043623160815218914;-0.015771947130012037;-0.00052231910477644353;-0.0059777472775860048]
      mask Display: e = 0.06;c1 = [120 150 230]/255;c2 = ([120 150 230]+0)/383;c3 = ([120 150 230]+128)/383;patch([0 1 1 0],[0 0 1 1],c1);patch([0 1 1 1-e 1-e 0+e],[0 0 1 1-e 0+e 0+e],c2);patch([0 0 1 1-e 0+e 0+e],[0 1 1 1-e 1-e 0+e],c3);plot([0 1 1 0 0],[0 0 1 1 0]);disp('Weights');
  "IW{1,2}(4,:)'" : Constant  Value=[-0.002561709904900874;0.051985039369039206;-0.026805050164739493;-0.0020744948180745175;0.042038321450945028;-0.025013537449072577;-0.0012398418620378029;0.033455721283894978;-0.023265622050217774;-0.00037113071725495422;0.026126400977093001;-0.021546345480203573;0.00083749953893930715;0.020122695548489489;-0.019917531482554322;0.0020786676233834644;0.015345334246164362;-0.018308076963373377;0.0034105206670790892;0.011693212286381299;-0.016784641738870551;0.0046661010403993858;0.0091111905405659513;-0.015322174642261285;0.0056008487631159821;0.0073377368780378144;-0.013917489306641469;0.0064291464174650792;0.0062672252972719254;-0.012587502836611289;0.0069575973245403645;0.0056587421928572324;-0.011330146559703222;0.0072442806975291079;0.0053676155681317006;-0.010123675067115845;0.0074197221497438182;0.0052850732935716266;-0.0090135351631428998;0.0071427505977573235;0.0052649616811593983;-0.0079162235194284551;0.0069010226940091676;0.0051150878767780997;-0.0068599995587133632;0.0066214230683530823;0.0048469936057280033;-0.0058510433418899853;0.0062180442228611946;0.0043647775874788739;-0.00488683947019524;0.0062475880585540176;0.0036438927221591;-0.0039356473032771538;0.0062394890186985349;0.0027160206979886937;-0.0029801709292729965;0.0065115592587869763;0.0016337155362715057;-0.0020815125594575248;0.00697737637414555;0.0004365635164495673;-0.0011770297123586328;0.0074707497967337012;-0.00087087313617048665;-0.00026879577332025495;0.0083702461775788713;-0.0021589759584111304;0.0006691132292261727;0.009158763648828127;-0.0034899405620055822;0.001573269010951208;0.0099820038980260092;-0.0047714357499309776;0.002497631744129908;0.011049187550682505;-0.0060392846708018331;0.0034059754518659859;0.011861548052627274;-0.0073185916051157762;0.0042924780387184856;0.012381466471740359;-0.00862492990884005;0.0052168046036146559;0.012849040094245617;-0.010127622999013177;0.0061392373558598109;0.011671778440313524;-0.011908808413391982;0.0070667646794730279]
      mask Display: e = 0.06;c1 = [120 150 230]/255;c2 = ([120 150 230]+0)/383;c3 = ([120 150 230]+128)/383;patch([0 1 1 0],[0 0 1 1],c1);patch([0 1 1 1-e 1-e 0+e],[0 0 1 1-e 0+e 0+e],c2);patch([0 0 1 1-e 0+e 0+e],[0 1 1 1-e 1-e 0+e],c3);plot([0 1 1 0 0],[0 0 1 1 0]);disp('Weights');
  "IW{1,2}(5,:)'" : Constant  Value=[0.037791593062023413;-0.077179434144811557;0.1044579637096902;0.036499249534754356;-0.04628075099093408;0.087681795524257838;0.034183976372743688;-0.021616525801156607;0.072104305615964939;0.034221587584454746;-0.002558177874225037;0.057731073981237842;0.032282942478084803;0.011562463794433018;0.044649484114990055;0.031474961756947854;0.021539136900392577;0.032833566468652015;0.030940588124845177;0.028053366136114193;0.02233251578460892;0.029345815059271547;0.03154521684232816;0.01309242393805368;0.029936335137279453;0.032644877567542488;0.0050979513376325346;0.028434036517099474;0.031689515372609882;-0.0016728664332432861;0.027789993797982571;0.029160267493305431;-0.0072397124677422448;0.02769454550527372;0.025473255707656219;-0.011656302289593534;0.025797909238908096;0.020934149630762251;-0.01499972999031176;0.026674936528987354;0.015797737596526935;-0.017247052418981054;0.02516460735210347;0.010346968828624112;-0.018529054747688851;0.024161403199454975;0.004792592129842229;-0.018881827346942558;0.024177627806202855;-0.00070453956878620727;-0.01835095457630875;0.022026679744769143;-0.0058199118084967579;-0.016999530565434077;0.022755092504432292;-0.010615882578770646;-0.014908518581418988;0.021628005234271205;-0.014720427759821344;-0.012099228124992978;0.020545480426328207;-0.018046042320733036;-0.0086226163419384633;0.021160953398463227;-0.020472811812747366;-0.0045654488271615603;0.01897947581970888;-0.02173385120610364;2.5588654097182335e-05;0.019988762065065429;-0.021654979669117384;0.0050932687587812416;0.020212415509449039;-0.019836236290383807;0.010560283906940778;0.016504475606535767;-0.016001589771848918;0.016439743607986848;0.016233152250411907;-0.0096596140071691997;0.02256403009247275;0.0091262805301225158;-0.00021723372043078786;0.028969690083678962;-0.0010680794224446463;0.013219543746700211;0.035486850645141704;-0.0093236563546136263;0.031207632886139407;0.042112006791117693]
      mask Display: e = 0.06;c1 = [120 150 230]/255;c2 = ([120 150 230]+0)/383;c3 = ([120 150 230]+128)/383;patch([0 1 1 0],[0 0 1 1],c1);patch([0 1 1 1-e 1-e 0+e],[0 0 1 1-e 0+e 0+e],c2);patch([0 0 1 1-e 0+e 0+e],[0 1 1 1-e 1-e 0+e],c3);plot([0 1 1 0 0],[0 0 1 1 0]);disp('Weights');
  "IW{1,2}(6,:)'" : Constant  Value=[-0.012835036788656533;0.078205401803860139;-0.069837453441485009;-0.010516227347881739;0.049436988435585819;-0.055852271414594673;-0.008000081335758278;0.027068498951633286;-0.042983494712621903;-0.0075185559256293289;0.010165246401295755;-0.031291482826682107;-0.0055388174676032345;-0.0020642596904269809;-0.020764769525618461;-0.0052217189214175596;-0.010540953939054999;-0.011469887832900297;-0.0045996021980605276;-0.016107533037193304;-0.0033646045506743501;-0.0041331453991476476;-0.019146070803193499;0.0035843758614775853;-0.0049733433041610504;-0.020356472229904828;0.0094515152800087841;-0.0045752519700079626;-0.02004633072498133;0.01421743311922182;-0.0050461633010047205;-0.018743864059529915;0.018051152712774313;-0.0058079095495780358;-0.016719940838173471;0.02098281350957636;-0.0052997660986676002;-0.014313854825990572;0.023121364998285925;-0.0068439931939410633;-0.01168775942160597;0.024509932667654537;-0.0067587249211306802;-0.0090719859088243884;0.025266973894570249;-0.0068709743594332672;-0.006474170446647832;0.025519036513852646;-0.0077370881727736917;-0.0040899470292561167;0.025267400367707801;-0.0070814696399539769;-0.0020820776298985867;0.024644595791196336;-0.0080413825302598912;-0.00016071437510110586;0.023692746178242741;-0.0077533603097144762;0.0015143109366047513;0.02251991128847184;-0.0074688545083794041;0.0029836694908992223;0.0210854403846144;-0.0077905220088997033;0.0043428529707211149;0.019555165752864576;-0.0058277476776772081;0.0055432097259395328;0.017880332316970449;-0.0063264420715206148;0.0064401275053752377;0.016143659464677922;-0.0052578940472996051;0.0069823219286863627;0.014382157736700768;-0.0029326612270651124;0.0070881786500543321;0.012575338588351173;-0.0027465912586317519;0.0064843227028833651;0.010772248562450317;-0.0019136731024228287;0.0045327559502105165;0.0090128134644445867;-0.0038407516306337257;-7.9296544337014653e-05;0.0073435735614875161;-0.0083316810251060063;-0.0078174942713188575;0.0057916778811200123]
      mask Display: e = 0.06;c1 = [120 150 230]/255;c2 = ([120 150 230]+0)/383;c3 = ([120 150 230]+128)/383;patch([0 1 1 0],[0 0 1 1],c1);patch([0 1 1 1-e 1-e 0+e],[0 0 1 1-e 0+e 0+e],c2);patch([0 0 1 1-e 0+e 0+e],[0 1 1 1-e 1-e 0+e],c3);plot([0 1 1 0 0],[0 0 1 1 0]);disp('Weights');
  "IW{1,2}(7,:)'" : Constant  Value=[-0.010046513237993498;-0.061836978802332021;-0.017597684248942244;-0.0082422023504158809;-0.055439263628782223;-0.013890228636180856;-0.007086635710827599;-0.048905551023665443;-0.010457991402986946;-0.0058325099966170559;-0.042409725294305492;-0.0072541300567199336;-0.0048397430981406619;-0.036108252393437408;-0.0043324775084829853;-0.0041345410758898337;-0.030087296348149859;-0.0016432960049855248;-0.0033239378243375109;-0.024455033368828448;0.00076246097415920118;-0.0029655912285282801;-0.019342727171694357;0.0029544019545176413;-0.0021907484947766738;-0.014723730073927303;0.0049156452536388805;-0.0014415524867522182;-0.010607313618266593;0.0066535901539584606;-0.00068936642588823241;-0.0068579276068936081;0.008139138442412373;0.0004315273561503725;-0.0035957916898106059;0.009407101183180477;0.0013716690138185221;-0.00065669881536488503;0.01046790484796069;0.0029046312301535802;0.0019365568129470255;0.011295483918085533;0.0043771295089622296;0.0042295281727613718;0.011944704457216173;0.0058978228635650238;0.0062921239341541067;0.012412553566786808;0.0078156551006058044;0.0081278769688686338;0.012677580315265545;0.009245027252723163;0.0097725810389074907;0.012772333891952458;0.011015327819771676;0.01109352633632585;0.012682212052876384;0.012575250760876873;0.012092006954948102;0.012400426765536727;0.014013508338820849;0.012675609860526852;0.011995956433376304;0.015532262406650286;0.012792254976713447;0.011445327107272814;0.016733281713129596;0.012393327257546398;0.010781004371097719;0.018128552605293394;0.011291630887981142;0.0099960216782434951;0.019835070768702848;0.0094187696466658671;0.0091045986441444862;0.021906863707879708;0.006625258408058712;0.0081081018047581537;0.025359442100743659;0.0028511205161923432;0.007050088062820664;0.031896858032419644;-0.0021131612111944054;0.0059699282067433822;0.041128520001425889;-0.0083008636162178098;0.0048440494328095551;0.058182600112877028;-0.015699056450110039;0.0037313958390941394]
      mask Display: e = 0.06;c1 = [120 150 230]/255;c2 = ([120 150 230]+0)/383;c3 = ([120 150 230]+128)/383;patch([0 1 1 0],[0 0 1 1],c1);patch([0 1 1 1-e 1-e 0+e],[0 0 1 1-e 0+e 0+e],c2);patch([0 0 1 1-e 0+e 0+e],[0 1 1 1-e 1-e 0+e],c3);plot([0 1 1 0 0],[0 0 1 1 0]);disp('Weights');
  Mux : Mux  Inputs=7
      mask Display: e = 0.06;c1 = [120 150 230]/255;c2 = ([120 150 230]+0)/383;c3 = ([120 150 230]+128)/383;patch([0 1 1 0],[0 0 1 1],c1);patch([0 1 1 1-e 1-e 0+e],[0 0 1 1-e 0+e 0+e],c2);patch([0 0 1 1-e 0+e 0+e],[0 1 1 1-e 1-e 0+e],c3);plot([0 1 1 0 0],[0 0 1 1 0]);disp('Mux');
  dotprod{1..7} (7 alike) : neural/Weight Functions/dotprod
  "iz{1,2}" : Outport
      mask Display: e = 0.06;c1 = [120 230 180]/255;c2 = ([120 230 180]+0)/(256+128);c3 = ([120 230 180]+128)/(256+128);patch([0 1 1 0],[0 0 1 1],c1);patch([0 1 1 1-e 1-e 0+e],[0 0 1 1-e 0+e 0+e],c2);patch([0 0 1 1-e 0+e 0+e],[0 1 1 1-e 1-e 0+e],c3);plot([0 1 1 0 0],[0 0 1 1 0]);
  wires:
  "IW{1,2}(1,:)'"/1 -> dotprod1/1
  "pd{1,2}"/1 -> dotprod1/2, dotprod2/2, dotprod3/2, dotprod4/2, dotprod5/2, dotprod6/2, dotprod7/2
  dotprod1/1 -> Mux/1
  "IW{1,2}(2,:)'"/1 -> dotprod2/1
  dotprod2/1 -> Mux/2
  "IW{1,2}(3,:)'"/1 -> dotprod3/1
  dotprod3/1 -> Mux/3
  "IW{1,2}(4,:)'"/1 -> dotprod4/1
  dotprod4/1 -> Mux/4
  "IW{1,2}(5,:)'"/1 -> dotprod5/1
  dotprod5/1 -> Mux/5
  "IW{1,2}(6,:)'"/1 -> dotprod6/1
  dotprod6/1 -> Mux/6
  "IW{1,2}(7,:)'"/1 -> dotprod7/1
  dotprod7/1 -> Mux/7
  Mux/1 -> "iz{1,2}"/1
